simulink model "diff_drive_staticFB_sim"  (R2018b)
settings: Solver=VariableStepAuto  StartTime=0.0  StopTime=489.5  RelTol=1e-3
values from neighbouring files (symbols this model uses):
  theta0 = atan2(ppval(fnder(sy,1), 0), ppval(fnder(sx,1), 0))    [diff_drive_staticFB.m]
  x0 = xwp(1)    [diff_drive_staticFB.m]
  y0 = ywp(1)    [diff_drive_staticFB.m]
undefined symbols (not defined in the file or in its folder): breaks, xc, xdc, xddc, yc, ydc, yddc
libraries: simulink x1
settings Model: Creator=olivier  LastModifiedBy=olivier
settings SolverCC: ZeroCrossAlgorithm=Adaptive
settings DebuggingCC: MaskedZcDiagnostic=none

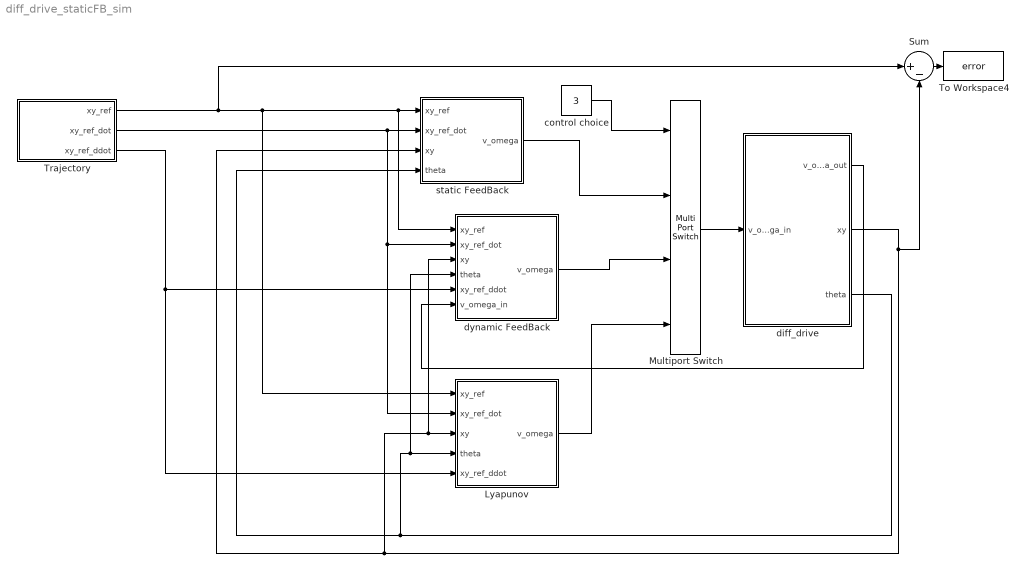
== system diff_drive_staticFB_sim ==
  Lyapunov : Subsystem
  Multiport Switch : MultiPortSwitch
  Sum : Sum  Inputs=|+-
  To Workspace4 : ToWorkspace  VariableName=error  SampleTime=-1
      settings: Save2DSignal=2-D array (concatenate along first dimension)
  Trajectory : Subsystem  TreatAsAtomicUnit=on  mask{time_scale=1}
      mask prompts: time_scale "time scale"
  control choice : Constant  Value=3
  diff_drive : Subsystem  mask{x0=x0, y0=y0, theta0=theta0, base=0.5, base_error=0, radius=0.2, radius_error=0, omega_max=80}
      mask prompts: base_error "Base error in percent"; radius_error "Radius error in percent"; omega_max "Wheel Max Velocity"
  dynamic FeedBack : Subsystem
  static FeedBack : Subsystem
  wires:
  Trajectory/1(xy_ref) -> Lyapunov/1(xy_ref), dynamic FeedBack/1(xy_ref), static FeedBack/1(xy_ref), Sum/1
  diff_drive/2(xy) -> Sum/2, dynamic FeedBack/3(xy), Lyapunov/3(xy), static FeedBack/3(xy)
  diff_drive/3(theta) -> dynamic FeedBack/4(theta), Lyapunov/4(theta), static FeedBack/4(theta)
  Trajectory/2(xy_ref_dot) -> Lyapunov/2(xy_ref_dot), dynamic FeedBack/2(xy_ref_dot), static FeedBack/2(xy_ref_dot)
  Sum/1 -> To Workspace4/1
  static FeedBack/1(v_omega) -> Multiport Switch/2
  Multiport Switch/1 -> diff_drive/1(v_omega_in)
  control choice/1 -> Multiport Switch/1
  Trajectory/3(xy_ref_ddot) -> Lyapunov/5(xy_ref_ddot), dynamic FeedBack/5(xy_ref_ddot)
  Lyapunov/1(v_omega) -> Multiport Switch/4
  dynamic FeedBack/1(v_omega) -> Multiport Switch/3
  diff_drive/1(v_omega_out) -> dynamic FeedBack/6(v_omega_in)

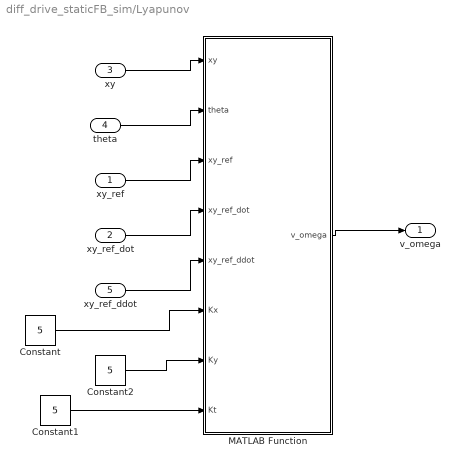
== system diff_drive_staticFB_sim/Lyapunov ==
  xy_ref : Inport
  xy_ref_dot : Inport  Port=2
  xy : Inport  Port=3
  theta : Inport  Port=4
  xy_ref_ddot : Inport  Port=5
  Constant : Constant  Value=5
  Constant1 : Constant  Value=5
  Constant2 : Constant  Value=5
  MATLAB Function : MATLAB Function  TreatAsAtomicUnit=on
  v_omega : Outport
  wires:
  theta/1 -> MATLAB Function/2(theta)
  xy/1 -> MATLAB Function/1(xy)
  xy_ref_ddot/1 -> MATLAB Function/5(xy_ref_ddot)
  xy_ref_dot/1 -> MATLAB Function/4(xy_ref_dot)
  xy_ref/1 -> MATLAB Function/3(xy_ref)
  MATLAB Function/1(v_omega) -> v_omega/1
  Constant/1 -> MATLAB Function/6(Kx)
  Constant1/1 -> MATLAB Function/8(Kt)
  Constant2/1 -> MATLAB Function/7(Ky)

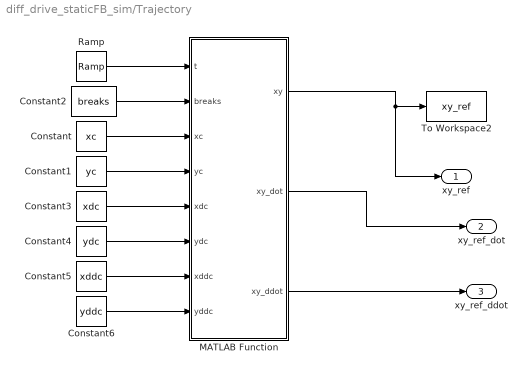
== system diff_drive_staticFB_sim/Trajectory ==
  Constant : Constant  Value=xc  VectorParams1D=off
  Constant1 : Constant  Value=yc  VectorParams1D=off
  Constant2 : Constant  Value=breaks  VectorParams1D=off
  Constant3 : Constant  Value=xdc  VectorParams1D=off
  Constant4 : Constant  Value=ydc  VectorParams1D=off
  Constant5 : Constant  Value=xddc  VectorParams1D=off
  Constant6 : Constant  Value=yddc  VectorParams1D=off
  MATLAB Function : MATLAB Function  TreatAsAtomicUnit=on
  Ramp : simulink/Sources/Ramp  slope=time_scale  start=0  InitialOutput=0
  To Workspace2 : ToWorkspace  VariableName=xy_ref  SampleTime=-1
      settings: Save2DSignal=2-D array (concatenate along first dimension)
  xy_ref : Outport
  xy_ref_dot : Outport  Port=2
  xy_ref_ddot : Outport  Port=3
  wires:
  Ramp/1 -> MATLAB Function/1(t)
  MATLAB Function/1(xy) -> xy_ref/1, To Workspace2/1
  Constant3/1 -> MATLAB Function/5(xdc)
  Constant4/1 -> MATLAB Function/6(ydc)
  Constant/1 -> MATLAB Function/3(xc)
  Constant2/1 -> MATLAB Function/2(breaks)
  Constant1/1 -> MATLAB Function/4(yc)
  Constant5/1 -> MATLAB Function/7(xddc)
  Constant6/1 -> MATLAB Function/8(yddc)
  MATLAB Function/3(xy_ddot) -> xy_ref_ddot/1
  MATLAB Function/2(xy_dot) -> xy_ref_dot/1

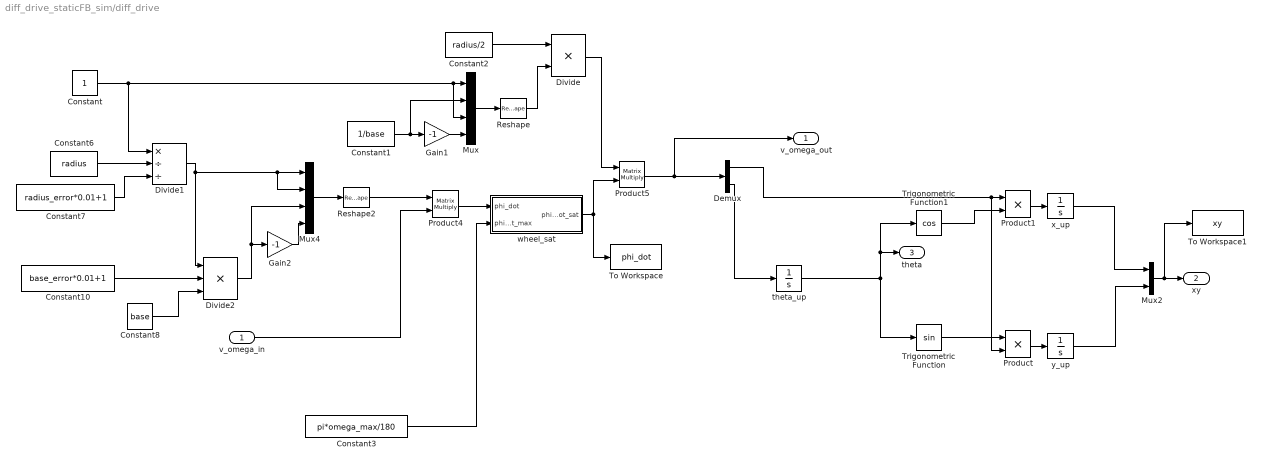
== system diff_drive_staticFB_sim/diff_drive ==
  v_omega_in : Inport
  Constant : Constant
  Constant1 : Constant  Value=1/base
  Constant10 : Constant  Value=base_error*0.01+1
  Constant2 : Constant  Value=radius/2
  Constant3 : Constant  Value=pi*omega_max/180
  Constant6 : Constant  Value=radius
  Constant7 : Constant  Value=radius_error*0.01+1
  Constant8 : Constant  Value=base
  Demux : Demux  Outputs=2
  Divide : Product  Inputs=**
  Divide1 : Product  Inputs=*//
  Divide2 : Product  Inputs=***
  Gain1 : Gain  Gain=-1
  Gain2 : Gain  Gain=-1
  Mux : Mux
  Mux2 : Mux  Inputs=2
  Mux4 : Mux
  Product : Product
  Product1 : Product
  Product4 : Product  Multiplication=Matrix(*)
  Product5 : Product  Multiplication=Matrix(*)
  Reshape : Reshape  OutputDimensionality=Customize  OutputDimensions=[2,2]
  Reshape2 : Reshape  OutputDimensionality=Customize  OutputDimensions=[2,2]
  To Workspace : ToWorkspace  VariableName=phi_dot  SampleTime=-1
      settings: Save2DSignal=2-D array (concatenate along first dimension)
  To Workspace1 : ToWorkspace  VariableName=xy  SampleTime=-1
      settings: Save2DSignal=2-D array (concatenate along first dimension)
  Trigonometric Function : Trigonometry
  Trigonometric Function1 : Trigonometry  Operator=cos
  theta_up : Integrator  InitialCondition=theta0
  wheel_sat : Subsystem
  x_up : Integrator  InitialCondition=x0
  y_up : Integrator  InitialCondition=y0
  v_omega_out : Outport
  xy : Outport  Port=2
  theta : Outport  Port=3
  wires:
  theta_up/1 -> theta/1, Trigonometric Function1/1, Trigonometric Function/1
  Trigonometric Function1/1 -> Product1/2
  Trigonometric Function/1 -> Product/1
  Product/1 -> y_up/1
  Product1/1 -> x_up/1
  x_up/1 -> Mux2/1
  Constant/1 -> Divide1/1, Mux/3, Mux/1
  Constant1/1 -> Gain1/1, Mux/2
  Mux/1 -> Reshape/1
  Constant2/1 -> Divide/1
  Divide/1 -> Product5/1
  Product4/1 -> wheel_sat/1(phi_dot)
  Constant3/1 -> wheel_sat/2(phi_dot_max)
  Product5/1 -> v_omega_out/1, Demux/1
  Demux/1 -> Product/2, Product1/1
  Demux/2 -> theta_up/1
  y_up/1 -> Mux2/2
  wheel_sat/1(phi_dot_sat) -> To Workspace/1, Product5/2
  Reshape2/1 -> Product4/1
  Gain1/1 -> Mux/4
  Mux4/1 -> Reshape2/1
  Constant6/1 -> Divide1/2
  Constant7/1 -> Divide1/3
  Divide1/1 -> Mux4/2, Mux4/1, Divide2/1
  Divide2/1 -> Mux4/3, Gain2/1
  Gain2/1 -> Mux4/4
  Mux2/1 -> To Workspace1/1, xy/1
  Constant8/1 -> Divide2/3
  Constant10/1 -> Divide2/2
  Reshape/1 -> Divide/2
  v_omega_in/1 -> Product4/2

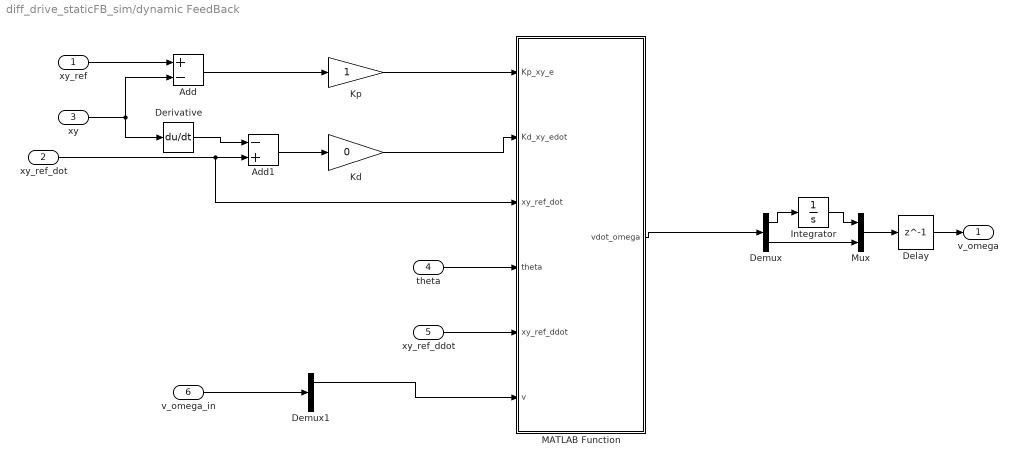
== system diff_drive_staticFB_sim/dynamic FeedBack ==
  xy_ref : Inport
  xy_ref_dot : Inport  Port=2
  xy : Inport  Port=3
  theta : Inport  Port=4
  xy_ref_ddot : Inport  Port=5
  v_omega_in : Inport  Port=6
  Add : Sum  Inputs=+-
  Add1 : Sum  Inputs=-+
  Delay : Delay  DelayLength=1  InitialCondition=0
  Demux : Demux  Outputs=2
  Demux1 : Demux  Outputs=2
  Derivative : Derivative
  Integrator : Integrator
  Kd : Gain  Gain=0
  Kp : Gain
  MATLAB Function : MATLAB Function  TreatAsAtomicUnit=on
  Mux : Mux  Inputs=2
  v_omega : Outport
  wires:
  theta/1 -> MATLAB Function/4(theta)
  xy_ref/1 -> Add/1
  xy/1 -> Derivative/1, Add/2
  Add/1 -> Kp/1
  xy_ref_dot/1 -> Add1/2, MATLAB Function/3(xy_ref_dot)
  Derivative/1 -> Add1/1
  Add1/1 -> Kd/1
  Demux/2 -> Mux/2
  Demux/1 -> Integrator/1
  Integrator/1 -> Mux/1
  Mux/1 -> Delay/1
  MATLAB Function/1(vdot_omega) -> Demux/1
  xy_ref_ddot/1 -> MATLAB Function/5(xy_ref_ddot)
  Kp/1 -> MATLAB Function/1(Kp_xy_e)
  Kd/1 -> MATLAB Function/2(Kd_xy_edot)
  v_omega_in/1 -> Demux1/1
  Demux1/1 -> MATLAB Function/6(v)
  Delay/1 -> v_omega/1

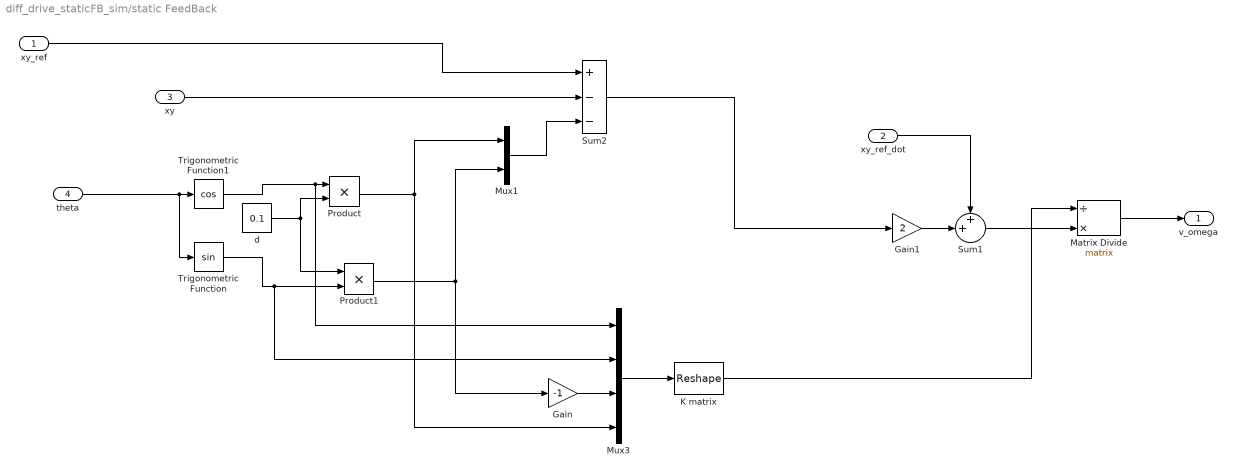
== system diff_drive_staticFB_sim/static FeedBack ==
  xy_ref : Inport
  xy_ref_dot : Inport  Port=2
  xy : Inport  Port=3
  theta : Inport  Port=4
  Gain : Gain  Gain=-1
  Gain1 : Gain  Gain=2
  K matrix : Reshape  OutputDimensionality=Customize  OutputDimensions=[2,2]
  Matrix Divide : Product  Inputs=/*  Multiplication=Matrix(*)
  Mux1 : Mux  Inputs=2
  Mux3 : Mux
  Product : Product
  Product1 : Product
  Sum1 : Sum  Inputs=++|
  Sum2 : Sum  Inputs=+--
  Trigonometric Function : Trigonometry
  Trigonometric Function1 : Trigonometry  Operator=cos
  d : Constant  Value=0.1
  v_omega : Outport
  wires:
  Product/1 -> Mux1/1, Mux3/4
  Trigonometric Function/1 -> Mux3/2, Product1/2
  Gain/1 -> Mux3/3
  Trigonometric Function1/1 -> Mux3/1, Product/1
  Mux3/1 -> K matrix/1
  Product1/1 -> Mux1/2, Gain/1
  d/1 -> Product1/1, Product/2
  Sum1/1 -> Matrix Divide/2
  Gain1/1 -> Sum1/2
  xy_ref_dot/1 -> Sum1/1
  xy_ref/1 -> Sum2/1
  xy/1 -> Sum2/2
  Mux1/1 -> Sum2/3
  Sum2/1 -> Gain1/1
  K matrix/1 -> Matrix Divide/1
  theta/1 -> Trigonometric Function/1, Trigonometric Function1/1
  Matrix Divide/1 -> v_omega/1

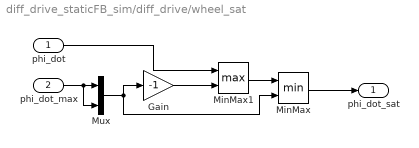
== system diff_drive_staticFB_sim/diff_drive/wheel_sat ==
  phi_dot : Inport
  phi_dot_max : Inport  Port=2
  Gain : Gain  Gain=-1
  MinMax : MinMax  Inputs=2
  MinMax1 : MinMax  Function=max  Inputs=2
  Mux : Mux  Inputs=2
  phi_dot_sat : Outport
  wires:
  Gain/1 -> MinMax1/2
  MinMax/1 -> phi_dot_sat/1
  phi_dot_max/1 -> Mux/2, Mux/1
  phi_dot/1 -> MinMax1/1
  MinMax1/1 -> MinMax/1
  Mux/1 -> MinMax/2, Gain/1

== matlab function diff_drive_staticFB_sim/dynamic FeedBack/MATLAB Function ==
  data: Kp_xy_e input; vdot_omega output; Kd_xy_edot input; xy_ref_dot input; theta input; xy_ref_ddot input; v input
function vdot_omega = dyn_FB(Kp_xy_e, Kd_xy_edot, xy_ref_dot, theta, xy_ref_ddot, v)

c = cos(theta);
s = sin(theta);

if abs(v) < 1e-3
    v = c * xy_ref_dot(1) + s * xy_ref_dot(2);
end
Finv = [c s; -s/v c/v];


vdot_omega = Finv * (xy_ref_ddot + Kd_xy_edot + Kp_xy_e);

== matlab function diff_drive_staticFB_sim/Trajectory/MATLAB Function ==
  data: xy output; t input; breaks input; xc input; yc input; xy_dot output; xy_ddot output; xdc input; ydc input; xddc input; yddc input
function [xy, xy_dot, xy_ddot] = reference(t, breaks, xc, yc, xdc, ydc, xddc, yddc)

sx = mkpp(breaks, xc);
sy = mkpp(breaks, yc);


if t > sx.breaks(end)
    t = sx.breaks(end);
    xy_dot = [0; 0];
    xy_ddot = [0; 0];
else
    xy_dot = [ppval(mkpp(breaks, xdc), t); ppval(mkpp(breaks, ydc), t)];
    xy_ddot = [ppval(mkpp(breaks, xddc), t); ppval(mkpp(breaks, yddc), t)];
end
xy = [ppval(sx, t); ppval(sy, t)];

== matlab function diff_drive_staticFB_sim/Lyapunov/MATLAB Function ==
  data: xy input; theta input; v_omega output; xy_ref input; xy_ref_dot input; xy_ref_ddot input; Kx input; Ky input; Kt input
function v_omega = lyapunov(xy, theta, xy_ref, xy_ref_dot, xy_ref_ddot, Kx, Ky, Kt)

c = cos(theta);
s = sin(theta);

% get position error in robot frame
xe = c * (xy_ref(1) - xy(1)) + s * (xy_ref(2) - xy(2));
ye = -s * (xy_ref(1) - xy(1)) + c * (xy_ref(2) - xy(2));
te = mod(atan2(xy_ref_dot(2), xy_ref_dot(1)) - theta + pi, 2*pi) - pi;

vref = c*xy_ref_dot(1) + s*xy_ref_dot(2);

if vref ~= 0
    wref = (xy_ref_dot(1) * xy_ref_ddot(2) - xy_ref_dot(2) * xy_ref_ddot(1))/vref^2;
else
   wref = 0; 
end


v_omega = [vref*cos(te) + Kx*xe ;wref + Ky*ye*vref*sinc(te) + Kt*te];
